simulink model "QuaterCar_Model"  (R2018b)
settings: Solver=VariableStepAuto  StartTime=0.0  StopTime=10.0  RelTol=1e-3
values from neighbouring files (symbols this model uses):
  cs =     [SetCoefficients.m]
  g = 9.81    [SetCoefficients_FC.m]
  ks =     [SetCoefficients.m]    (also in SetCoefficients_FC.m = 20000)
  m1 = 250    [SetCoefficients.m]    (also in SetCoefficients_FC.m)
settings Model: Creator=joebe  LastModifiedBy=joebe

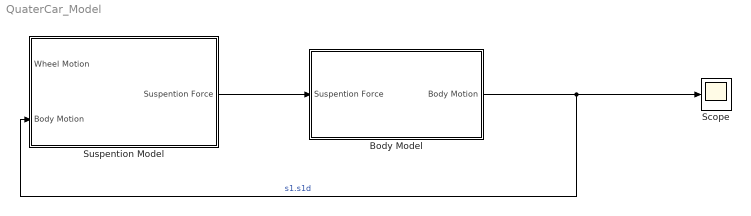
== system QuaterCar_Model ==
  Body Model : Subsystem
  Scope : Scope
  Suspention Model : Subsystem
  wires:
  Suspention Model/1(Suspention Force) -> Body Model/1("Suspention Force ")
  Body Model/1(Body Motion) -> Suspention Model/2(Body Motion), Scope/1  "s1.s1d"

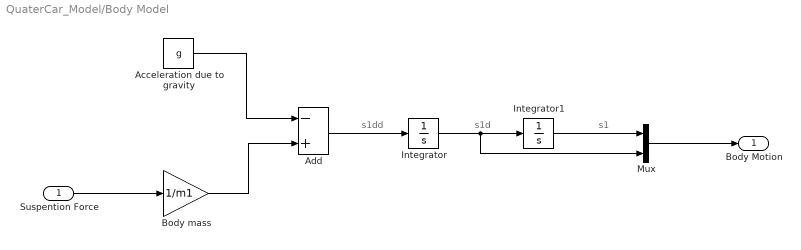
== system QuaterCar_Model/Body Model ==
  note: s1d
  note: s1
  note: s1dd
  "Suspention Force " : Inport
  Acceleration due to gravity : Constant  Value=g
  Add : Sum  Inputs=-+
  Body mass : Gain  Gain=1/m1
  Integrator : Integrator
  Integrator1 : Integrator
  Mux : Mux  Inputs=2
  Body Motion : Outport
  wires:
  Body mass/1 -> Add/2
  Integrator/1 -> Mux/2, Integrator1/1
  Add/1 -> Integrator/1
  Acceleration due to gravity/1 -> Add/1
  Integrator1/1 -> Mux/1
  "Suspention Force "/1 -> Body mass/1
  Mux/1 -> Body Motion/1

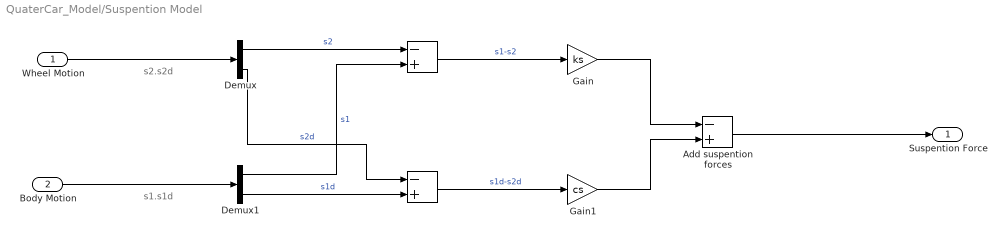
== system QuaterCar_Model/Suspention Model ==
  note: s1.s1d
  note: s2.s2d
  Wheel Motion : Inport
  Body Motion : Inport  Port=2
  " " : Sum  Inputs=-+
  " " : Sum  Inputs=-+
  Add suspention forces : Sum  Inputs=-+
  Demux : Demux  Outputs=2
  Demux1 : Demux  Outputs=2
  Gain : Gain  Gain=ks
  Gain1 : Gain  Gain=cs
  Suspention Force : Outport
  wires:
  Demux1/2 -> " "/2  "s1d"
  " "/1 -> Gain/1  "s1-s2"
  Demux1/1 -> " "/2  "s1"
  Gain1/1 -> Add suspention forces/2
  Gain/1 -> Add suspention forces/1
  Demux/1 -> " "/1  "s2"
  Demux/2 -> " "/1  "s2d"
  Body Motion/1 -> Demux1/1
  " "/1 -> Gain1/1  "s1d-s2d"
  Add suspention forces/1 -> Suspention Force/1
  Wheel Motion/1 -> Demux/1
